simulink model "Model_turn"  (R2024a)
settings: Solver=VariableStepAuto  StartTime=0.0  StopTime=100  MaxStep=0.1  RelTol=1e-3
values from neighbouring files (symbols this model uses):
  c_SMA = 837.36    [params.m]
  Fmax_SMA = 10    [params.m]
  h_SMA = .3    (= 0.3)    [params.m]
  k_gn = m*g/0.01    (= 9810)    [contact3D_params.m]
  k_gt = m*g/0.1    (= 981)    [contact3D_params.m]
  m = 10    [contact3D_params.m]
  m_SMA = 0.0025    [params.m]
  max_SMA_Energy_J = 150    [params.m]
  mu_slide = 0.8    [contact3D_params.m]
  mu_stick = 0.9    [contact3D_params.m]
  n_segs = 10    [params.m]
  PWM_max = 0.35    [params.m]
  R_SMA = .08    (= 0.08)    [params.m]
  r_SMA2limb = 0.009    [params.m]
  swing_angle = swing_angles(i)    [params.m]
  T_amb = 23    [params.m]
  V_0 = 7    [params.m]
  v_gn_max = 0.03    [contact3D_params.m]
  v_gt_max = 0.03    [contact3D_params.m]
  vLimit = 0.01    [contact3D_params.m]
undefined symbols (not defined in the file or in its folder): Newton, Raphson, X, Y, Z
libraries: sm_lib x225, nesl_utility x185, simulink x24, simulink_extras x6
(part 15 of 16)

== system Model_turn/LIMB 1: Front LEFT/Limb 1/Right Ball Contact/3D Contact/Kinetic Friction Model ==
  note: Kinetic Friction Model
  note: Footpoint Determiner
  note: Sliding Limit Detector
  note: Normal Ground Friction
  note: Tangential Ground Friction
  vel [m/s m/s m/s] : Inport
  pos [m m m] : Inport  Port=2
  RefPt [m m m] : Inport  Port=3
  nVec [m m m] : Inport  Port=4
  Enable : EnablePort  StatesWhenEnabling=reset  ZeroCross=off
  Constant : Constant  Value=vLimit
  Constant1 : Constant  Value=[0 0 0 1]'
  Demux : Demux  Outputs=[3 1]
  FixPt Relational Operator : RelationalOperator  Operator=>  OutDataTypeStr=boolean  ZeroCross=off  InputSameDT=off
  Gain3 : Gain  Gain=k_gn
  Gain4 : Gain  Gain=1/v_gn_max
  Memory : Memory
  Mux1 : Mux  Inputs=2
  Mux2 : Mux  Inputs=2
  Negative : simulink/Logic and Bit Operations/Compare To Zero  relop=<  OutDataTypeStr=boolean
  Normal Axis Ground Force : Fcn  Expr="u(1)  *  (1-u(2)) * (u(2)<1)"
  Product : Product  RndMeth=Zero
  Product1 : Product  RndMeth=Zero
  Sum : Sum  Inputs=|+-
  Switch : Switch  Criteria=u2 > Threshold  Threshold=0.9*vLimit  SaturateOnIntegerOverflow=off  InputSameDT=off
      settings: AttributesFormatString=>%<Threshold>?
  Vector Norm : Subsystem
  d_n : DotProduct  OutDataTypeStr=Inherit: Inherit via internal rule
  qnVec : Sum  Inputs=-+
  reverse direction : Gain  Gain=-1
  sliding friction coefficient : Gain  Gain=mu_slide
  tVec : Product  Inputs=*/  RndMeth=Zero
  v_n : DotProduct  OutDataTypeStr=Inherit: Inherit via internal rule
  v_nVec : Product  RndMeth=Zero
  v_tVec : Sum  Inputs=-+|
  RefPtFP [m m m] : Outport  InitialOutput=[0 0 0]
      settings: AttributesFormatString=initial = '%<InitialOutput>'\nwhen disabled = '%<OutputWhenDisabled>'
  posFP [m m m] : Outport  Port=2  InitialOutput=[0 0 0]
      settings: AttributesFormatString=initial = '%<InitialOutput>'\nwhen disabled = '%<OutputWhenDisabled>'
  nVec FP [m m m] : Outport  Port=3  InitialOutput=0
      settings: AttributesFormatString=initial = '%<InitialOutput>'\nwhen disabled = '%<OutputWhenDisabled>'
  Stiction! : Outport  Port=4  OutputWhenDisabled=reset  InitialOutput=0
      settings: AttributesFormatString=initial = '%<InitialOutput>'\nwhen disabled = '%<OutputWhenDisabled>'
  F_t Slide [N N N] : Outport  Port=5  OutputWhenDisabled=reset  InitialOutput=[0 0 0]
      settings: AttributesFormatString=initial = '%<InitialOutput>'\nwhen disabled = '%<OutputWhenDisabled>'
  F_n Slide [N N N] : Outport  Port=6  OutputWhenDisabled=reset  InitialOutput=[0 0 0]
      settings: AttributesFormatString=initial = '%<InitialOutput>'\nwhen disabled = '%<OutputWhenDisabled>'
  wires:
  Normal Axis Ground Force/1 -> sliding friction coefficient/1, Product1/2
  Product/1 -> F_t Slide [N N N]/1
  FixPt Relational Operator/1 -> Stiction!/1
  Memory/1 -> FixPt Relational Operator/2
  Negative/1 -> FixPt Relational Operator/1, Memory/1
  Vector Norm/1(norm) -> Sum/1, Switch/2, Mux2/2
  Sum/1 -> Negative/1
  Constant/1 -> Sum/2
  Mux1/1 -> Normal Axis Ground Force/1
  Gain3/1 -> Mux1/1
  Gain4/1 -> Mux1/2
  nVec [m m m]/1 -> v_n/1, v_nVec/2, d_n/2, Product1/1, nVec FP [m m m]/1
  d_n/1 -> Gain3/1
  vel [m/s m/s m/s]/1 -> v_n/2, v_tVec/2
  v_n/1 -> Gain4/1, v_nVec/1
  v_nVec/1 -> v_tVec/1
  v_tVec/1 -> Vector Norm/1(vec), Mux2/1
  sliding friction coefficient/1 -> Product/1
  reverse direction/1 -> Product/2
  Product1/1 -> F_n Slide [N N N]/1
  tVec/1 -> reverse direction/1
  Constant1/1 -> Switch/3
  Mux2/1 -> Switch/1
  Switch/1 -> Demux/1
  Demux/2 -> tVec/2
  Demux/1 -> tVec/1
  pos [m m m]/1 -> posFP [m m m]/1, qnVec/1
  qnVec/1 -> d_n/1
  RefPt [m m m]/1 -> qnVec/2, RefPtFP [m m m]/1

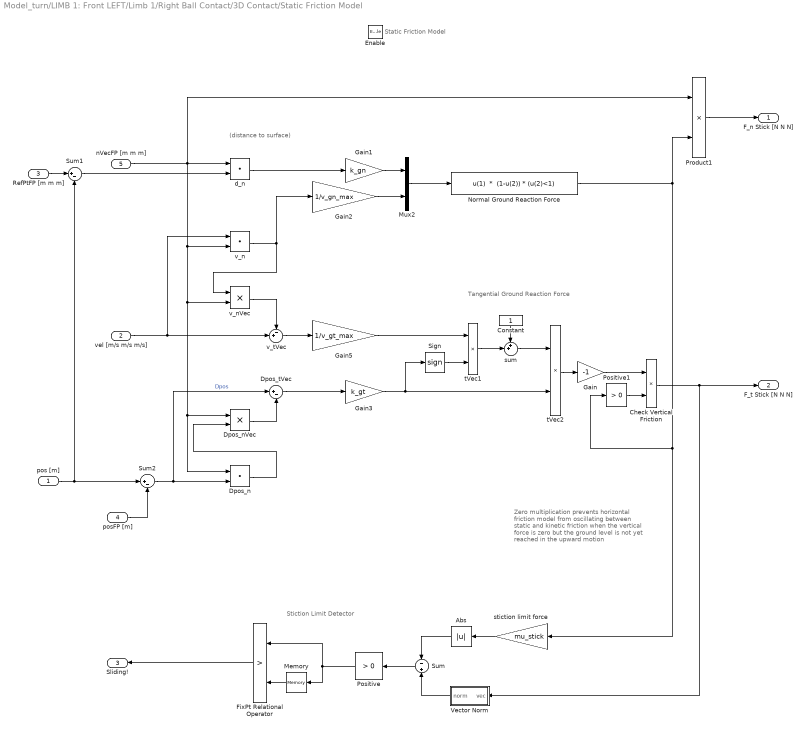
== system Model_turn/LIMB 1: Front LEFT/Limb 1/Right Ball Contact/3D Contact/Static Friction Model ==
  note: Stiction Limit Detector
  note: Static Friction Model
  note: Zero multiplication prevents
      | horizontal friction model from
      | oscillating between static and kinetic
      | friction when the vertical force is zero but
      | the ground level is not yet reached
      | in the upward motion
  note: (distance to
      | surface)
  note: Tangential Ground Reaction Force
  pos [m] : Inport
  vel [m/s m/s m/s] : Inport  Port=2
  RefPtFP [m m m] : Inport  Port=3
  posFP [m] : Inport  Port=4
  nVecFP [m m m] : Inport  Port=5
  Enable : EnablePort  StatesWhenEnabling=reset  ZeroCross=off
  Abs : Abs  SaturateOnIntegerOverflow=off
  Check Vertical Friction : Product  RndMeth=Zero
  Constant : Constant
  Dpos_n : DotProduct  OutDataTypeStr=Inherit: Inherit via internal rule
  Dpos_nVec : Product  RndMeth=Zero
  Dpos_tVec : Sum  Inputs=|+-
  FixPt Relational Operator : RelationalOperator  Operator=>  OutDataTypeStr=boolean  ZeroCross=off  InputSameDT=off
  Gain : Gain  Gain=-1
  Gain1 : Gain  Gain=k_gn
  Gain2 : Gain  Gain=1/v_gn_max
  Gain3 : Gain  Gain=k_gt
  Gain5 : Gain  Gain=1/v_gt_max
  Memory : Memory
  Mux2 : Mux  Inputs=2
  Normal Ground Reaction Force : Fcn  Expr="u(1)  *  (1-u(2)) * (u(2)<1)"
  Positive : simulink/Logic and Bit Operations/Compare To Zero  relop=>  OutDataTypeStr=boolean
  Positive1 : simulink/Logic and Bit Operations/Compare To Zero  relop=>  OutDataTypeStr=boolean
  Product1 : Product  RndMeth=Zero
  Sign : Signum  ZeroCross=off
  Sum : Sum  Inputs=-+
  Sum1 : Sum  Inputs=|+-
  Sum2 : Sum  Inputs=|+-
  Vector Norm : Subsystem
  d_n : DotProduct  OutDataTypeStr=Inherit: Inherit via internal rule
  stiction limit force : Gain  Gain=mu_stick
  sum : Sum  Inputs=++|
  tVec1 : Product  Inputs=**  RndMeth=Zero
  tVec2 : Product  Inputs=**  RndMeth=Zero
  v_n : DotProduct  OutDataTypeStr=Inherit: Inherit via internal rule
  v_nVec : Product  RndMeth=Zero
  v_tVec : Sum  Inputs=-+|
  F_n Stick [N N N] : Outport  OutputWhenDisabled=reset  InitialOutput=[0 0 0]
      settings: AttributesFormatString=initial = '%<InitialOutput>'\nwhen disabled = '%<OutputWhenDisabled>'
  F_t Stick [N N N] : Outport  Port=2  OutputWhenDisabled=reset  InitialOutput=[0 0 0]
      settings: AttributesFormatString=when disabled: %<OutputWhenDisabled>\ninitial: %<InitialOutput>
  Sliding! : Outport  Port=3  OutputWhenDisabled=reset  InitialOutput=0
      settings: AttributesFormatString=when disabled: %<OutputWhenDisabled>\ninitial: %<InitialOutput>
  wires:
  Sum/1 -> Positive/1
  Memory/1 -> FixPt Relational Operator/2
  Positive/1 -> FixPt Relational Operator/1, Memory/1
  FixPt Relational Operator/1 -> Sliding!/1
  Abs/1 -> Sum/1
  stiction limit force/1 -> Abs/1
  Positive1/1 -> Check Vertical Friction/2
  Check Vertical Friction/1 -> Vector Norm/1(vec), F_t Stick [N N N]/1
  Normal Ground Reaction Force/1 -> Product1/2, stiction limit force/1, Positive1/1
  Mux2/1 -> Normal Ground Reaction Force/1
  Gain1/1 -> Mux2/1
  Gain2/1 -> Mux2/2
  nVecFP [m m m]/1 -> d_n/1, v_n/2, Dpos_n/1, Dpos_nVec/1, v_nVec/2, Product1/1
  d_n/1 -> Gain1/1
  vel [m/s m/s m/s]/1 -> v_tVec/2, v_n/1
  v_n/1 -> v_nVec/1, Gain2/1
  v_nVec/1 -> v_tVec/1
  v_tVec/1 -> Gain5/1
  Product1/1 -> F_n Stick [N N N]/1
  pos [m]/1 -> Sum2/1, Sum1/2
  posFP [m]/1 -> Sum2/2
  Sum2/1 -> Dpos_n/2, Dpos_tVec/1  "Dpos"
  Dpos_n/1 -> Dpos_nVec/2
  Dpos_nVec/1 -> Dpos_tVec/2
  Dpos_tVec/1 -> Gain3/1
  Gain3/1 -> Sign/1, tVec2/2
  Sign/1 -> tVec1/2
  tVec1/1 -> sum/2
  Constant/1 -> sum/1
  sum/1 -> tVec2/1
  tVec2/1 -> Gain/1
  Gain/1 -> Check Vertical Friction/1
  Vector Norm/1(norm) -> Sum/2
  RefPtFP [m m m]/1 -> Sum1/1
  Sum1/1 -> d_n/2
  Gain5/1 -> tVec1/1

== system Model_turn/LIMB 1: Front RIGHT/Limb 1/Right Ball Contact/3D Contact/Friction Switch ==
  note: Static/Kinetic Friction Switch
  Slide! : Inport
  Stick! : Inport  Port=2
  Memory : Memory
  S-R Flip-Flop : simulink_extras/Flip Flops/S-R Flip-Flop  initial_condition=0
  Terminator : Terminator
  Stiction : Outport
  wires:
  S-R Flip-Flop/1 -> Memory/1
  S-R Flip-Flop/2 -> Terminator/1
  Stick!/1 -> S-R Flip-Flop/1
  Slide!/1 -> S-R Flip-Flop/2
  Memory/1 -> Stiction/1

== system Model_turn/LIMB 1: Front RIGHT/Limb 1/Right Ball Contact/3D Contact/Kinetic Friction Model ==
  note: Kinetic Friction Model
  note: Footpoint Determiner
  note: Sliding Limit Detector
  note: Normal Ground Friction
  note: Tangential Ground Friction
  vel [m/s m/s m/s] : Inport
  pos [m m m] : Inport  Port=2
  RefPt [m m m] : Inport  Port=3
  nVec [m m m] : Inport  Port=4
  Enable : EnablePort  StatesWhenEnabling=reset  ZeroCross=off
  Constant : Constant  Value=vLimit
  Constant1 : Constant  Value=[0 0 0 1]'
  Demux : Demux  Outputs=[3 1]
  FixPt Relational Operator : RelationalOperator  Operator=>  OutDataTypeStr=boolean  ZeroCross=off  InputSameDT=off
  Gain3 : Gain  Gain=k_gn
  Gain4 : Gain  Gain=1/v_gn_max
  Memory : Memory
  Mux1 : Mux  Inputs=2
  Mux2 : Mux  Inputs=2
  Negative : simulink/Logic and Bit Operations/Compare To Zero  relop=<  OutDataTypeStr=boolean
  Normal Axis Ground Force : Fcn  Expr="u(1)  *  (1-u(2)) * (u(2)<1)"
  Product : Product  RndMeth=Zero
  Product1 : Product  RndMeth=Zero
  Sum : Sum  Inputs=|+-
  Switch : Switch  Criteria=u2 > Threshold  Threshold=0.9*vLimit  SaturateOnIntegerOverflow=off  InputSameDT=off
      settings: AttributesFormatString=>%<Threshold>?
  Vector Norm : Subsystem
  d_n : DotProduct  OutDataTypeStr=Inherit: Inherit via internal rule
  qnVec : Sum  Inputs=-+
  reverse direction : Gain  Gain=-1
  sliding friction coefficient : Gain  Gain=mu_slide
  tVec : Product  Inputs=*/  RndMeth=Zero
  v_n : DotProduct  OutDataTypeStr=Inherit: Inherit via internal rule
  v_nVec : Product  RndMeth=Zero
  v_tVec : Sum  Inputs=-+|
  RefPtFP [m m m] : Outport  InitialOutput=[0 0 0]
      settings: AttributesFormatString=initial = '%<InitialOutput>'\nwhen disabled = '%<OutputWhenDisabled>'
  posFP [m m m] : Outport  Port=2  InitialOutput=[0 0 0]
      settings: AttributesFormatString=initial = '%<InitialOutput>'\nwhen disabled = '%<OutputWhenDisabled>'
  nVec FP [m m m] : Outport  Port=3  InitialOutput=0
      settings: AttributesFormatString=initial = '%<InitialOutput>'\nwhen disabled = '%<OutputWhenDisabled>'
  Stiction! : Outport  Port=4  OutputWhenDisabled=reset  InitialOutput=0
      settings: AttributesFormatString=initial = '%<InitialOutput>'\nwhen disabled = '%<OutputWhenDisabled>'
  F_t Slide [N N N] : Outport  Port=5  OutputWhenDisabled=reset  InitialOutput=[0 0 0]
      settings: AttributesFormatString=initial = '%<InitialOutput>'\nwhen disabled = '%<OutputWhenDisabled>'
  F_n Slide [N N N] : Outport  Port=6  OutputWhenDisabled=reset  InitialOutput=[0 0 0]
      settings: AttributesFormatString=initial = '%<InitialOutput>'\nwhen disabled = '%<OutputWhenDisabled>'
  wires:
  Normal Axis Ground Force/1 -> sliding friction coefficient/1, Product1/2
  Product/1 -> F_t Slide [N N N]/1
  FixPt Relational Operator/1 -> Stiction!/1
  Memory/1 -> FixPt Relational Operator/2
  Negative/1 -> FixPt Relational Operator/1, Memory/1
  Vector Norm/1(norm) -> Sum/1, Switch/2, Mux2/2
  Sum/1 -> Negative/1
  Constant/1 -> Sum/2
  Mux1/1 -> Normal Axis Ground Force/1
  Gain3/1 -> Mux1/1
  Gain4/1 -> Mux1/2
  nVec [m m m]/1 -> v_n/1, v_nVec/2, d_n/2, Product1/1, nVec FP [m m m]/1
  d_n/1 -> Gain3/1
  vel [m/s m/s m/s]/1 -> v_n/2, v_tVec/2
  v_n/1 -> Gain4/1, v_nVec/1
  v_nVec/1 -> v_tVec/1
  v_tVec/1 -> Vector Norm/1(vec), Mux2/1
  sliding friction coefficient/1 -> Product/1
  reverse direction/1 -> Product/2
  Product1/1 -> F_n Slide [N N N]/1
  tVec/1 -> reverse direction/1
  Constant1/1 -> Switch/3
  Mux2/1 -> Switch/1
  Switch/1 -> Demux/1
  Demux/2 -> tVec/2
  Demux/1 -> tVec/1
  pos [m m m]/1 -> posFP [m m m]/1, qnVec/1
  qnVec/1 -> d_n/1
  RefPt [m m m]/1 -> qnVec/2, RefPtFP [m m m]/1

== system Model_turn/LIMB 1: Front RIGHT/Limb 1/Right Ball Contact/3D Contact/Static Friction Model ==
  note: Stiction Limit Detector
  note: Static Friction Model
  note: Zero multiplication prevents
      | horizontal friction model from
      | oscillating between static and kinetic
      | friction when the vertical force is zero but
      | the ground level is not yet reached
      | in the upward motion
  note: (distance to
      | surface)
  note: Tangential Ground Reaction Force
  pos [m] : Inport
  vel [m/s m/s m/s] : Inport  Port=2
  RefPtFP [m m m] : Inport  Port=3
  posFP [m] : Inport  Port=4
  nVecFP [m m m] : Inport  Port=5
  Enable : EnablePort  StatesWhenEnabling=reset  ZeroCross=off
  Abs : Abs  SaturateOnIntegerOverflow=off
  Check Vertical Friction : Product  RndMeth=Zero
  Constant : Constant
  Dpos_n : DotProduct  OutDataTypeStr=Inherit: Inherit via internal rule
  Dpos_nVec : Product  RndMeth=Zero
  Dpos_tVec : Sum  Inputs=|+-
  FixPt Relational Operator : RelationalOperator  Operator=>  OutDataTypeStr=boolean  ZeroCross=off  InputSameDT=off
  Gain : Gain  Gain=-1
  Gain1 : Gain  Gain=k_gn
  Gain2 : Gain  Gain=1/v_gn_max
  Gain3 : Gain  Gain=k_gt
  Gain5 : Gain  Gain=1/v_gt_max
  Memory : Memory
  Mux2 : Mux  Inputs=2
  Normal Ground Reaction Force : Fcn  Expr="u(1)  *  (1-u(2)) * (u(2)<1)"
  Positive : simulink/Logic and Bit Operations/Compare To Zero  relop=>  OutDataTypeStr=boolean
  Positive1 : simulink/Logic and Bit Operations/Compare To Zero  relop=>  OutDataTypeStr=boolean
  Product1 : Product  RndMeth=Zero
  Sign : Signum  ZeroCross=off
  Sum : Sum  Inputs=-+
  Sum1 : Sum  Inputs=|+-
  Sum2 : Sum  Inputs=|+-
  Vector Norm : Subsystem
  d_n : DotProduct  OutDataTypeStr=Inherit: Inherit via internal rule
  stiction limit force : Gain  Gain=mu_stick
  sum : Sum  Inputs=++|
  tVec1 : Product  Inputs=**  RndMeth=Zero
  tVec2 : Product  Inputs=**  RndMeth=Zero
  v_n : DotProduct  OutDataTypeStr=Inherit: Inherit via internal rule
  v_nVec : Product  RndMeth=Zero
  v_tVec : Sum  Inputs=-+|
  F_n Stick [N N N] : Outport  OutputWhenDisabled=reset  InitialOutput=[0 0 0]
      settings: AttributesFormatString=initial = '%<InitialOutput>'\nwhen disabled = '%<OutputWhenDisabled>'
  F_t Stick [N N N] : Outport  Port=2  OutputWhenDisabled=reset  InitialOutput=[0 0 0]
      settings: AttributesFormatString=when disabled: %<OutputWhenDisabled>\ninitial: %<InitialOutput>
  Sliding! : Outport  Port=3  OutputWhenDisabled=reset  InitialOutput=0
      settings: AttributesFormatString=when disabled: %<OutputWhenDisabled>\ninitial: %<InitialOutput>
  wires:
  Sum/1 -> Positive/1
  Memory/1 -> FixPt Relational Operator/2
  Positive/1 -> FixPt Relational Operator/1, Memory/1
  FixPt Relational Operator/1 -> Sliding!/1
  Abs/1 -> Sum/1
  stiction limit force/1 -> Abs/1
  Positive1/1 -> Check Vertical Friction/2
  Check Vertical Friction/1 -> Vector Norm/1(vec), F_t Stick [N N N]/1
  Normal Ground Reaction Force/1 -> Product1/2, stiction limit force/1, Positive1/1
  Mux2/1 -> Normal Ground Reaction Force/1
  Gain1/1 -> Mux2/1
  Gain2/1 -> Mux2/2
  nVecFP [m m m]/1 -> d_n/1, v_n/2, Dpos_n/1, Dpos_nVec/1, v_nVec/2, Product1/1
  d_n/1 -> Gain1/1
  vel [m/s m/s m/s]/1 -> v_tVec/2, v_n/1
  v_n/1 -> v_nVec/1, Gain2/1
  v_nVec/1 -> v_tVec/1
  v_tVec/1 -> Gain5/1
  Product1/1 -> F_n Stick [N N N]/1
  pos [m]/1 -> Sum2/1, Sum1/2
  posFP [m]/1 -> Sum2/2
  Sum2/1 -> Dpos_n/2, Dpos_tVec/1  "Dpos"
  Dpos_n/1 -> Dpos_nVec/2
  Dpos_nVec/1 -> Dpos_tVec/2
  Dpos_tVec/1 -> Gain3/1
  Gain3/1 -> Sign/1, tVec2/2
  Sign/1 -> tVec1/2
  tVec1/1 -> sum/2
  Constant/1 -> sum/1
  sum/1 -> tVec2/1
  tVec2/1 -> Gain/1
  Gain/1 -> Check Vertical Friction/1
  Vector Norm/1(norm) -> Sum/2
  RefPtFP [m m m]/1 -> Sum1/1
  Sum1/1 -> d_n/2
  Gain5/1 -> tVec1/1

== system Model_turn/LIMB 1: Back LEFT/Limb 1/Right Ball Contact/3D Contact/Kinetic Friction Model/Vector Norm ==
  vec : Inport
  Sqrt : Sqrt  OutputSignalType=real  AlgorithmType=Newton-Raphson
  Squares : Math  Operator=square  SignedPower=on  OutputSignalType=real
  Sum of Elements : Sum  Inputs=+
  norm : Outport
  wires:
  vec/1 -> Squares/1
  Sqrt/1 -> norm/1
  Sum of Elements/1 -> Sqrt/1
  Squares/1 -> Sum of Elements/1

== system Model_turn/LIMB 1: Back LEFT/Limb 1/Right Ball Contact/3D Contact/Static Friction Model/Vector Norm ==
  vec : Inport
  Sqrt : Sqrt  OutputSignalType=real  AlgorithmType=Newton-Raphson
  Squares : Math  Operator=square  SignedPower=on  OutputSignalType=real
  Sum of Elements : Sum  Inputs=+
  norm : Outport
  wires:
  vec/1 -> Squares/1
  Sqrt/1 -> norm/1
  Sum of Elements/1 -> Sqrt/1
  Squares/1 -> Sum of Elements/1

== system Model_turn/LIMB 1: Back RIGHT/Limb 1/Right Ball Contact/3D Contact/Kinetic Friction Model/Vector Norm ==
  vec : Inport
  Sqrt : Sqrt  OutputSignalType=real  AlgorithmType=Newton-Raphson
  Squares : Math  Operator=square  SignedPower=on  OutputSignalType=real
  Sum of Elements : Sum  Inputs=+
  norm : Outport
  wires:
  vec/1 -> Squares/1
  Sqrt/1 -> norm/1
  Sum of Elements/1 -> Sqrt/1
  Squares/1 -> Sum of Elements/1

== system Model_turn/LIMB 1: Back RIGHT/Limb 1/Right Ball Contact/3D Contact/Static Friction Model/Vector Norm ==
  vec : Inport
  Sqrt : Sqrt  OutputSignalType=real  AlgorithmType=Newton-Raphson
  Squares : Math  Operator=square  SignedPower=on  OutputSignalType=real
  Sum of Elements : Sum  Inputs=+
  norm : Outport
  wires:
  vec/1 -> Squares/1
  Sqrt/1 -> norm/1
  Sum of Elements/1 -> Sqrt/1
  Squares/1 -> Sum of Elements/1

== system Model_turn/LIMB 1: Center LEFT/Limb 1/Right Ball Contact/3D Contact/Kinetic Friction Model/Vector Norm ==
  vec : Inport
  Sqrt : Sqrt  OutputSignalType=real  AlgorithmType=Newton-Raphson
  Squares : Math  Operator=square  SignedPower=on  OutputSignalType=real
  Sum of Elements : Sum  Inputs=+
  norm : Outport
  wires:
  vec/1 -> Squares/1
  Sqrt/1 -> norm/1
  Sum of Elements/1 -> Sqrt/1
  Squares/1 -> Sum of Elements/1

== system Model_turn/LIMB 1: Center LEFT/Limb 1/Right Ball Contact/3D Contact/Static Friction Model/Vector Norm ==
  vec : Inport
  Sqrt : Sqrt  OutputSignalType=real  AlgorithmType=Newton-Raphson
  Squares : Math  Operator=square  SignedPower=on  OutputSignalType=real
  Sum of Elements : Sum  Inputs=+
  norm : Outport
  wires:
  vec/1 -> Squares/1
  Sqrt/1 -> norm/1
  Sum of Elements/1 -> Sqrt/1
  Squares/1 -> Sum of Elements/1

== system Model_turn/LIMB 1: Center RIGHT/Limb 1/Right Ball Contact/3D Contact/Kinetic Friction Model/Vector Norm ==
  vec : Inport
  Sqrt : Sqrt  OutputSignalType=real  AlgorithmType=Newton-Raphson
  Squares : Math  Operator=square  SignedPower=on  OutputSignalType=real
  Sum of Elements : Sum  Inputs=+
  norm : Outport
  wires:
  vec/1 -> Squares/1
  Sqrt/1 -> norm/1
  Sum of Elements/1 -> Sqrt/1
  Squares/1 -> Sum of Elements/1

== system Model_turn/LIMB 1: Center RIGHT/Limb 1/Right Ball Contact/3D Contact/Static Friction Model/Vector Norm ==
  vec : Inport
  Sqrt : Sqrt  OutputSignalType=real  AlgorithmType=Newton-Raphson
  Squares : Math  Operator=square  SignedPower=on  OutputSignalType=real
  Sum of Elements : Sum  Inputs=+
  norm : Outport
  wires:
  vec/1 -> Squares/1
  Sqrt/1 -> norm/1
  Sum of Elements/1 -> Sqrt/1
  Squares/1 -> Sum of Elements/1

== system Model_turn/LIMB 1: Front LEFT/Limb 1/Right Ball Contact/3D Contact/Kinetic Friction Model/Vector Norm ==
  vec : Inport
  Sqrt : Sqrt  OutputSignalType=real  AlgorithmType=Newton-Raphson
  Squares : Math  Operator=square  SignedPower=on  OutputSignalType=real
  Sum of Elements : Sum  Inputs=+
  norm : Outport
  wires:
  vec/1 -> Squares/1
  Sqrt/1 -> norm/1
  Sum of Elements/1 -> Sqrt/1
  Squares/1 -> Sum of Elements/1

== system Model_turn/LIMB 1: Front LEFT/Limb 1/Right Ball Contact/3D Contact/Static Friction Model/Vector Norm ==
  vec : Inport
  Sqrt : Sqrt  OutputSignalType=real  AlgorithmType=Newton-Raphson
  Squares : Math  Operator=square  SignedPower=on  OutputSignalType=real
  Sum of Elements : Sum  Inputs=+
  norm : Outport
  wires:
  vec/1 -> Squares/1
  Sqrt/1 -> norm/1
  Sum of Elements/1 -> Sqrt/1
  Squares/1 -> Sum of Elements/1

== system Model_turn/LIMB 1: Front RIGHT/Limb 1/Right Ball Contact/3D Contact/Kinetic Friction Model/Vector Norm ==
  vec : Inport
  Sqrt : Sqrt  OutputSignalType=real  AlgorithmType=Newton-Raphson
  Squares : Math  Operator=square  SignedPower=on  OutputSignalType=real
  Sum of Elements : Sum  Inputs=+
  norm : Outport
  wires:
  vec/1 -> Squares/1
  Sqrt/1 -> norm/1
  Sum of Elements/1 -> Sqrt/1
  Squares/1 -> Sum of Elements/1

== system Model_turn/LIMB 1: Front RIGHT/Limb 1/Right Ball Contact/3D Contact/Static Friction Model/Vector Norm ==
  vec : Inport
  Sqrt : Sqrt  OutputSignalType=real  AlgorithmType=Newton-Raphson
  Squares : Math  Operator=square  SignedPower=on  OutputSignalType=real
  Sum of Elements : Sum  Inputs=+
  norm : Outport
  wires:
  vec/1 -> Squares/1
  Sqrt/1 -> norm/1
  Sum of Elements/1 -> Sqrt/1
  Squares/1 -> Sum of Elements/1

== matlab function Model_turn/LIMB 1: Back RIGHT/Limb 1/MATLAB Function2 ==
  data: R input; roll_deg output; pitch_deg output; yaw_deg output
function [roll_deg, pitch_deg, yaw_deg] = orientation_to_plane_angles(R)
    roll = atan2(R(3,2), R(3,3));
    pitch = asin(-R(3,1));
    yaw = atan2(R(2,1), R(1,1));
    % Convert angles from radians to degrees
    roll_deg = rad2deg(roll);
    pitch_deg = rad2deg(pitch);
    yaw_deg = rad2deg(yaw);

end

== matlab function Model_turn/LIMB 1: Back RIGHT/Limb 1/SMA1 F(V)/F(T) ==
  data: T input; F output; Fmax_SMA input
function F = fcn(T, Fmax_SMA)

% INPUT: Temperature (C), max SMA force
% OUTPUT: Force [N]

% Based around T_transition = 90C

% THOS WHOLE RELATIONSHIP NEEDS IMPROVEMENT, LOOSELY BASED ON fig 6b from:
% https://link.springer.com/article/10.1007/s11340-024-01059-9 and 
% https://www.dynalloy.com/pdfs/TCF1140_2.pdf
if T>110
    F = Fmax_SMA;
elseif T>95
    F = Fmax_SMA - 0.2*Fmax_SMA * ((110-T)/15);
elseif T>85
    F = 0.8*Fmax_SMA - 0.55*Fmax_SMA * ((95-T)/10);
else
    F = 0.25*Fmax_SMA - 0.25*Fmax_SMA * ((85-T)/50);
end

== matlab function Model_turn/LIMB 1: Back RIGHT/Limb 1/SMA2 F(V)/F(T) ==
  data: T input; F output; Fmax_SMA input
function F = fcn(T, Fmax_SMA)

% INPUT: Temperature (C), max SMA force
% OUTPUT: Force [N]

% Based around T_transition = 90C

% THOS WHOLE RELATIONSHIP NEEDS IMPROVEMENT, LOOSELY BASED ON fig 6b from:
% https://link.springer.com/article/10.1007/s11340-024-01059-9 and 
% https://www.dynalloy.com/pdfs/TCF1140_2.pdf
if T>110
    F = Fmax_SMA;
elseif T>95
    F = Fmax_SMA - 0.2*Fmax_SMA * ((110-T)/15);
elseif T>85
    F = 0.8*Fmax_SMA - 0.55*Fmax_SMA * ((95-T)/10);
else
    F = 0.25*Fmax_SMA - 0.25*Fmax_SMA * ((85-T)/50);
end

== matlab function Model_turn/LIMB 1: Back RIGHT/Limb 1/SMA3 F(V)/F(T) ==
  data: T input; F output; Fmax_SMA input
function F = fcn(T, Fmax_SMA)

% INPUT: Temperature (C), max SMA force
% OUTPUT: Force [N]

% Based around T_transition = 90C

% THOS WHOLE RELATIONSHIP NEEDS IMPROVEMENT, LOOSELY BASED ON fig 6b from:
% https://link.springer.com/article/10.1007/s11340-024-01059-9 and 
% https://www.dynalloy.com/pdfs/TCF1140_2.pdf
if T>110
    F = Fmax_SMA;
elseif T>95
    F = Fmax_SMA - 0.2*Fmax_SMA * ((110-T)/15);
elseif T>85
    F = 0.8*Fmax_SMA - 0.55*Fmax_SMA * ((95-T)/10);
else
    F = 0.25*Fmax_SMA - 0.25*Fmax_SMA * ((85-T)/50);
end

== matlab function Model_turn/LIMB 1: Back RIGHT/Limb 1/SMA4 F(V)/F(T) ==
  data: T input; F output; Fmax_SMA input
function F = fcn(T, Fmax_SMA)

% INPUT: Temperature (C), max SMA force
% OUTPUT: Force [N]

% Based around T_transition = 90C

% THOS WHOLE RELATIONSHIP NEEDS IMPROVEMENT, LOOSELY BASED ON fig 6b from:
% https://link.springer.com/article/10.1007/s11340-024-01059-9 and 
% https://www.dynalloy.com/pdfs/TCF1140_2.pdf
if T>110
    F = Fmax_SMA;
elseif T>95
    F = Fmax_SMA - 0.2*Fmax_SMA * ((110-T)/15);
elseif T>85
    F = 0.8*Fmax_SMA - 0.55*Fmax_SMA * ((95-T)/10);
else
    F = 0.25*Fmax_SMA - 0.25*Fmax_SMA * ((85-T)/50);
end

== matlab function Model_turn/LIMB 1: Back RIGHT/PID CONTROLLER ==
  data: eX input; deX input; seX input; D1 output; eY input; D2 output; D3 output; D4 output; deY input; seY input; PWM_max input
function [D1, D2, D3, D4] = fcn(eX, deX, seX, eY, deY, seY, PWM_max)

    % INPUT: errors and derivatives about -x and -y axes, max PWM
    % OUTPUT: Duty Cycles:

    kp = 0.5;
    kd = 0;
    ki = 0.05;

    D1 = 0; D2 = 0; D3 = 0; D4 = 0;

    if eX > 0.5
        D1 = min((kp*eX + kd*deX + ki*seX), PWM_max);
    elseif eX < -0.5
        D2 = min((kp*-eX + kd*-deX + ki*-seX), PWM_max);
    end

    if eY > 0.5
        D3 = min((kp*eY + kd*deY + ki*seY), PWM_max);
    elseif eY < -0.5
        D4 = min((kp*-eY + kd*-deY + ki*-seY), PWM_max);
    end

== matlab function Model_turn/LIMB 1: Front LEFT/BANG-BANG CONTROLLER ==
  data: theta_X input; D1 output; theta_Y input; D2 output; D3 output; D4 output; Target_X input; Target_Y input; PWM_max input
function [D1, D2, D3, D4] = fcn(theta_X, theta_Y, Target_X, Target_Y, PWM_max)

    % INPUT: Rotations about -X and -Y axes, Target angles, max PWM
    % OUTPUT: Duty Cycles:
    %   D1: +X rotation
    %   D2: -X rotation
    %   D3: +Y rotation
    %   D4: -Y rotation

    X_err = Target_X - theta_X;
    Y_err = Target_Y - theta_Y;

    D1 = 0; D2 = 0; D3 = 0; D4 = 0;

    if X_err > 5
        D1 = PWM_max;
    elseif X_err > 1
        D1 = PWM_max / 1.5;
    elseif X_err < -5
        D2 = PWM_max;
    elseif X_err < -1
        D2 = PWM_max / 1.5;
    end

    if Y_err > 5
        D3 = PWM_max;
    elseif Y_err > 1
        D3 = PWM_max / 1.5;
    elseif Y_err < -5
        D4 = PWM_max;
    elseif Y_err < -1
        D4 = PWM_max / 1.5;
    end

== matlab function Model_turn/LIMB 1: Front LEFT/Limb 1/MATLAB Function1 ==
  data: R input; alpha_xz output; alpha_yz output; alpha_xy output
function [alpha_xz, alpha_yz, alpha_xy] = orientation_to_plane_angles(R)
% ORIENTATION_TO_PLANE_ANGLES Convert orientation to angle projections on XZ, YZ, XY planes
%   Inputs:
%       R - Rotation Matrix
%   Outputs:
%       alpha_xz - Angle in radians on the XZ-plane
%       alpha_yz - Angle in radians on the YZ-plane
%       alpha_xy - Angle in radians on the XY-plane
    
    % Define the local forward vector (local Z-axis)
    v_local = [0; 0; 1];
    
    % Transform to global coordinates
    v_global = R * v_local;
    
    % Projection onto XZ-plane
    v_xz = [v_global(1); 0; v_global(3)];
    alpha_xz = rad2deg(-(atan2(v_xz(3), v_xz(1)) - pi/2));
    
    % Projection onto YZ-plane
    v_yz = [0; v_global(2); v_global(3)];
    alpha_yz = rad2deg(atan2(v_yz(3), v_yz(2)) - pi/2);
    
    % Projection onto XY-plane
    v_xy = [v_global(1); v_global(2); 0];
    alpha_xy = rad2deg(atan2(v_xy(2), v_xy(1)) + pi/4);
end

== matlab function Model_turn/LIMB 1: Front LEFT/Limb 1/SMA1 F(V)/F(T) ==
  data: T input; F output; Fmax_SMA input
function F = fcn(T, Fmax_SMA)

% INPUT: Temperature (C), max SMA force
% OUTPUT: Force [N]

% Based around T_transition = 90C

% THOS WHOLE RELATIONSHIP NEEDS IMPROVEMENT, LOOSELY BASED ON fig 6b from:
% https://link.springer.com/article/10.1007/s11340-024-01059-9 and 
% https://www.dynalloy.com/pdfs/TCF1140_2.pdf
if T>110
    F = Fmax_SMA;
elseif T>95
    F = Fmax_SMA - 0.2*Fmax_SMA * ((110-T)/15);
elseif T>85
    F = 0.8*Fmax_SMA - 0.55*Fmax_SMA * ((95-T)/10);
else
    F = 0.25*Fmax_SMA - 0.25*Fmax_SMA * ((85-T)/50);
end

== matlab function Model_turn/LIMB 1: Front LEFT/Limb 1/SMA2 F(V)/F(T) ==
  data: T input; F output; Fmax_SMA input
function F = fcn(T, Fmax_SMA)

% INPUT: Temperature (C), max SMA force
% OUTPUT: Force [N]

% Based around T_transition = 90C

% THOS WHOLE RELATIONSHIP NEEDS IMPROVEMENT, LOOSELY BASED ON fig 6b from:
% https://link.springer.com/article/10.1007/s11340-024-01059-9 and 
% https://www.dynalloy.com/pdfs/TCF1140_2.pdf
if T>110
    F = Fmax_SMA;
elseif T>95
    F = Fmax_SMA - 0.2*Fmax_SMA * ((110-T)/15);
elseif T>85
    F = 0.8*Fmax_SMA - 0.55*Fmax_SMA * ((95-T)/10);
else
    F = 0.25*Fmax_SMA - 0.25*Fmax_SMA * ((85-T)/50);
end

== matlab function Model_turn/LIMB 1: Front LEFT/Limb 1/SMA3 F(V)/F(T) ==
  data: T input; F output; Fmax_SMA input
function F = fcn(T, Fmax_SMA)

% INPUT: Temperature (C), max SMA force
% OUTPUT: Force [N]

% Based around T_transition = 90C

% THOS WHOLE RELATIONSHIP NEEDS IMPROVEMENT, LOOSELY BASED ON fig 6b from:
% https://link.springer.com/article/10.1007/s11340-024-01059-9 and 
% https://www.dynalloy.com/pdfs/TCF1140_2.pdf
if T>110
    F = Fmax_SMA;
elseif T>95
    F = Fmax_SMA - 0.2*Fmax_SMA * ((110-T)/15);
elseif T>85
    F = 0.8*Fmax_SMA - 0.55*Fmax_SMA * ((95-T)/10);
else
    F = 0.25*Fmax_SMA - 0.25*Fmax_SMA * ((85-T)/50);
end

== matlab function Model_turn/LIMB 1: Front LEFT/Limb 1/SMA4 F(V)/F(T) ==
  data: T input; F output; Fmax_SMA input
function F = fcn(T, Fmax_SMA)

% INPUT: Temperature (C), max SMA force
% OUTPUT: Force [N]

% Based around T_transition = 90C

% THOS WHOLE RELATIONSHIP NEEDS IMPROVEMENT, LOOSELY BASED ON fig 6b from:
% https://link.springer.com/article/10.1007/s11340-024-01059-9 and 
% https://www.dynalloy.com/pdfs/TCF1140_2.pdf
if T>110
    F = Fmax_SMA;
elseif T>95
    F = Fmax_SMA - 0.2*Fmax_SMA * ((110-T)/15);
elseif T>85
    F = 0.8*Fmax_SMA - 0.55*Fmax_SMA * ((95-T)/10);
else
    F = 0.25*Fmax_SMA - 0.25*Fmax_SMA * ((85-T)/50);
end

== matlab function Model_turn/LIMB 1: Front LEFT/PID CONTROLLER ==
  data: eX input; deX input; seX input; D1 output; eY input; D2 output; D3 output; D4 output; deY input; seY input; PWM_max input
function [D1, D2, D3, D4] = fcn(eX, deX, seX, eY, deY, seY, PWM_max)

    % INPUT: errors and derivatives about -x and -y axes, max PWM
    % OUTPUT: Duty Cycles:

    kp = 0.5;
    kd = 0;
    ki = 0.05;

    D1 = 0; D2 = 0; D3 = 0; D4 = 0;

    if eX > 0.5
        D1 = min((kp*eX + kd*deX + ki*seX), PWM_max);
    elseif eX < -0.5
        D2 = min((kp*-eX + kd*-deX + ki*-seX), PWM_max);
    end

    if eY > 0.5
        D3 = min((kp*eY + kd*deY + ki*seY), PWM_max);
    elseif eY < -0.5
        D4 = min((kp*-eY + kd*-deY + ki*-seY), PWM_max);
    end

== matlab function Model_turn/LIMB 1: Back LEFT/BANG-BANG CONTROLLER ==
  data: theta_X input; D1 output; theta_Y input; D2 output; D3 output; D4 output; Target_X input; Target_Y input; PWM_max input
function [D1, D2, D3, D4] = fcn(theta_X, theta_Y, Target_X, Target_Y, PWM_max)

    % INPUT: Rotations about -X and -Y axes, Target angles, max PWM
    % OUTPUT: Duty Cycles:
    %   D1: +X rotation
    %   D2: -X rotation
    %   D3: +Y rotation
    %   D4: -Y rotation

    X_err = Target_X - theta_X;
    Y_err = Target_Y - theta_Y;

    D1 = 0; D2 = 0; D3 = 0; D4 = 0;

    if X_err > 5
        D1 = PWM_max;
    elseif X_err > 1
        D1 = PWM_max / 1.5;
    elseif X_err < -5
        D2 = PWM_max;
    elseif X_err < -1
        D2 = PWM_max / 1.5;
    end

    if Y_err > 5
        D3 = PWM_max;
    elseif Y_err > 1
        D3 = PWM_max / 1.5;
    elseif Y_err < -5
        D4 = PWM_max;
    elseif Y_err < -1
        D4 = PWM_max / 1.5;
    end

== matlab function Model_turn/LIMB 1: Back LEFT/Limb 1/MATLAB Function2 ==
  data: R input; roll_deg output; pitch_deg output; yaw_deg output
function [roll_deg, pitch_deg, yaw_deg] = orientation_to_plane_angles(R)
    roll = atan2(R(3,2), R(3,3));
    pitch = asin(-R(3,1));
    yaw = atan2(R(2,1), R(1,1));
    % Convert angles from radians to degrees
    roll_deg = rad2deg(roll);
    pitch_deg = rad2deg(pitch);
    yaw_deg = rad2deg(yaw);

end

== matlab function Model_turn/LIMB 1: Center LEFT/Limb 1/SMA2 F(V)/F(T) ==
  data: T input; F output; Fmax_SMA input
function F = fcn(T, Fmax_SMA)

% INPUT: Temperature (C), max SMA force
% OUTPUT: Force [N]

% Based around T_transition = 90C

% THOS WHOLE RELATIONSHIP NEEDS IMPROVEMENT, LOOSELY BASED ON fig 6b from:
% https://link.springer.com/article/10.1007/s11340-024-01059-9 and 
% https://www.dynalloy.com/pdfs/TCF1140_2.pdf
if T>110
    F = Fmax_SMA;
elseif T>95
    F = Fmax_SMA - 0.2*Fmax_SMA * ((110-T)/15);
elseif T>85
    F = 0.8*Fmax_SMA - 0.55*Fmax_SMA * ((95-T)/10);
else
    F = 0.25*Fmax_SMA - 0.25*Fmax_SMA * ((85-T)/50);
end

== matlab function Model_turn/LIMB 1: Back LEFT/Limb 1/SMA1 F(V)/F(T) ==
  data: T input; F output; Fmax_SMA input
function F = fcn(T, Fmax_SMA)

% INPUT: Temperature (C), max SMA force
% OUTPUT: Force [N]

% Based around T_transition = 90C

% THOS WHOLE RELATIONSHIP NEEDS IMPROVEMENT, LOOSELY BASED ON fig 6b from:
% https://link.springer.com/article/10.1007/s11340-024-01059-9 and 
% https://www.dynalloy.com/pdfs/TCF1140_2.pdf
if T>110
    F = Fmax_SMA;
elseif T>95
    F = Fmax_SMA - 0.2*Fmax_SMA * ((110-T)/15);
elseif T>85
    F = 0.8*Fmax_SMA - 0.55*Fmax_SMA * ((95-T)/10);
else
    F = 0.25*Fmax_SMA - 0.25*Fmax_SMA * ((85-T)/50);
end

== matlab function Model_turn/LIMB 1: Back LEFT/Limb 1/SMA2 F(V)/F(T) ==
  data: T input; F output; Fmax_SMA input
function F = fcn(T, Fmax_SMA)

% INPUT: Temperature (C), max SMA force
% OUTPUT: Force [N]

% Based around T_transition = 90C

% THOS WHOLE RELATIONSHIP NEEDS IMPROVEMENT, LOOSELY BASED ON fig 6b from:
% https://link.springer.com/article/10.1007/s11340-024-01059-9 and 
% https://www.dynalloy.com/pdfs/TCF1140_2.pdf
if T>110
    F = Fmax_SMA;
elseif T>95
    F = Fmax_SMA - 0.2*Fmax_SMA * ((110-T)/15);
elseif T>85
    F = 0.8*Fmax_SMA - 0.55*Fmax_SMA * ((95-T)/10);
else
    F = 0.25*Fmax_SMA - 0.25*Fmax_SMA * ((85-T)/50);
end

== matlab function Model_turn/LIMB 1: Back LEFT/Limb 1/SMA3 F(V)/F(T) ==
  data: T input; F output; Fmax_SMA input
function F = fcn(T, Fmax_SMA)

% INPUT: Temperature (C), max SMA force
% OUTPUT: Force [N]

% Based around T_transition = 90C

% THOS WHOLE RELATIONSHIP NEEDS IMPROVEMENT, LOOSELY BASED ON fig 6b from:
% https://link.springer.com/article/10.1007/s11340-024-01059-9 and 
% https://www.dynalloy.com/pdfs/TCF1140_2.pdf
if T>110
    F = Fmax_SMA;
elseif T>95
    F = Fmax_SMA - 0.2*Fmax_SMA * ((110-T)/15);
elseif T>85
    F = 0.8*Fmax_SMA - 0.55*Fmax_SMA * ((95-T)/10);
else
    F = 0.25*Fmax_SMA - 0.25*Fmax_SMA * ((85-T)/50);
end

== matlab function Model_turn/LIMB 1: Back LEFT/Limb 1/SMA4 F(V)/F(T) ==
  data: T input; F output; Fmax_SMA input
function F = fcn(T, Fmax_SMA)

% INPUT: Temperature (C), max SMA force
% OUTPUT: Force [N]

% Based around T_transition = 90C

% THOS WHOLE RELATIONSHIP NEEDS IMPROVEMENT, LOOSELY BASED ON fig 6b from:
% https://link.springer.com/article/10.1007/s11340-024-01059-9 and 
% https://www.dynalloy.com/pdfs/TCF1140_2.pdf
if T>110
    F = Fmax_SMA;
elseif T>95
    F = Fmax_SMA - 0.2*Fmax_SMA * ((110-T)/15);
elseif T>85
    F = 0.8*Fmax_SMA - 0.55*Fmax_SMA * ((95-T)/10);
else
    F = 0.25*Fmax_SMA - 0.25*Fmax_SMA * ((85-T)/50);
end

== matlab function Model_turn/LIMB 1: Back LEFT/PID CONTROLLER ==
  data: eX input; deX input; seX input; D1 output; eY input; D2 output; D3 output; D4 output; deY input; seY input; PWM_max input
function [D1, D2, D3, D4] = fcn(eX, deX, seX, eY, deY, seY, PWM_max)

    % INPUT: errors and derivatives about -x and -y axes, max PWM
    % OUTPUT: Duty Cycles:

    kp = 0.5;
    kd = 0;
    ki = 0.05;

    D1 = 0; D2 = 0; D3 = 0; D4 = 0;

    if eX > 0.5
        D1 = min((kp*eX + kd*deX + ki*seX), PWM_max);
    elseif eX < -0.5
        D2 = min((kp*-eX + kd*-deX + ki*-seX), PWM_max);
    end

    if eY > 0.5
        D3 = min((kp*eY + kd*deY + ki*seY), PWM_max);
    elseif eY < -0.5
        D4 = min((kp*-eY + kd*-deY + ki*-seY), PWM_max);
    end

== matlab function Model_turn/LIMB 1: Center RIGHT/BANG-BANG CONTROLLER ==
  data: theta_X input; D1 output; theta_Y input; D2 output; D3 output; D4 output; Target_X input; Target_Y input; PWM_max input
function [D1, D2, D3, D4] = fcn(theta_X, theta_Y, Target_X, Target_Y, PWM_max)

    % INPUT: Rotations about -X and -Y axes, Target angles, max PWM
    % OUTPUT: Duty Cycles:
    %   D1: +X rotation
    %   D2: -X rotation
    %   D3: +Y rotation
    %   D4: -Y rotation

    X_err = Target_X - theta_X;
    Y_err = Target_Y - theta_Y;

    D1 = 0; D2 = 0; D3 = 0; D4 = 0;

    if X_err > 5
        D1 = PWM_max;
    elseif X_err > 1
        D1 = PWM_max / 1.5;
    elseif X_err < -5
        D2 = PWM_max;
    elseif X_err < -1
        D2 = PWM_max / 1.5;
    end

    if Y_err > 5
        D3 = PWM_max;
    elseif Y_err > 1
        D3 = PWM_max / 1.5;
    elseif Y_err < -5
        D4 = PWM_max;
    elseif Y_err < -1
        D4 = PWM_max / 1.5;
    end

== matlab function Model_turn/LIMB 1: Center RIGHT/Limb 1/MATLAB Function2 ==
  data: R input; roll_deg output; pitch_deg output; yaw_deg output
function [roll_deg, pitch_deg, yaw_deg] = orientation_to_plane_angles(R)
    roll = atan2(R(3,2), R(3,3));
    pitch = asin(-R(3,1));
    yaw = atan2(R(2,1), R(1,1));
    % Convert angles from radians to degrees
    roll_deg = rad2deg(roll);
    pitch_deg = rad2deg(pitch);
    yaw_deg = rad2deg(yaw);

end

== matlab function Model_turn/LIMB 1: Center RIGHT/Limb 1/SMA1 F(V)/F(T) ==
  data: T input; F output; Fmax_SMA input
function F = fcn(T, Fmax_SMA)

% INPUT: Temperature (C), max SMA force
% OUTPUT: Force [N]

% Based around T_transition = 90C

% THOS WHOLE RELATIONSHIP NEEDS IMPROVEMENT, LOOSELY BASED ON fig 6b from:
% https://link.springer.com/article/10.1007/s11340-024-01059-9 and 
% https://www.dynalloy.com/pdfs/TCF1140_2.pdf
if T>110
    F = Fmax_SMA;
elseif T>95
    F = Fmax_SMA - 0.2*Fmax_SMA * ((110-T)/15);
elseif T>85
    F = 0.8*Fmax_SMA - 0.55*Fmax_SMA * ((95-T)/10);
else
    F = 0.25*Fmax_SMA - 0.25*Fmax_SMA * ((85-T)/50);
end

== matlab function Model_turn/LIMB 1: Center LEFT/Limb 1/SMA1 F(V)/F(T) ==
  data: T input; F output; Fmax_SMA input
function F = fcn(T, Fmax_SMA)

% INPUT: Temperature (C), max SMA force
% OUTPUT: Force [N]

% Based around T_transition = 90C

% THOS WHOLE RELATIONSHIP NEEDS IMPROVEMENT, LOOSELY BASED ON fig 6b from:
% https://link.springer.com/article/10.1007/s11340-024-01059-9 and 
% https://www.dynalloy.com/pdfs/TCF1140_2.pdf
if T>110
    F = Fmax_SMA;
elseif T>95
    F = Fmax_SMA - 0.2*Fmax_SMA * ((110-T)/15);
elseif T>85
    F = 0.8*Fmax_SMA - 0.55*Fmax_SMA * ((95-T)/10);
else
    F = 0.25*Fmax_SMA - 0.25*Fmax_SMA * ((85-T)/50);
end

== matlab function Model_turn/LIMB 1: Center RIGHT/Limb 1/SMA2 F(V)/F(T) ==
  data: T input; F output; Fmax_SMA input
function F = fcn(T, Fmax_SMA)

% INPUT: Temperature (C), max SMA force
% OUTPUT: Force [N]

% Based around T_transition = 90C

% THOS WHOLE RELATIONSHIP NEEDS IMPROVEMENT, LOOSELY BASED ON fig 6b from:
% https://link.springer.com/article/10.1007/s11340-024-01059-9 and 
% https://www.dynalloy.com/pdfs/TCF1140_2.pdf
if T>110
    F = Fmax_SMA;
elseif T>95
    F = Fmax_SMA - 0.2*Fmax_SMA * ((110-T)/15);
elseif T>85
    F = 0.8*Fmax_SMA - 0.55*Fmax_SMA * ((95-T)/10);
else
    F = 0.25*Fmax_SMA - 0.25*Fmax_SMA * ((85-T)/50);
end

== matlab function Model_turn/LIMB 1: Center RIGHT/Limb 1/SMA3 F(V)/F(T) ==
  data: T input; F output; Fmax_SMA input
function F = fcn(T, Fmax_SMA)

% INPUT: Temperature (C), max SMA force
% OUTPUT: Force [N]

% Based around T_transition = 90C

% THOS WHOLE RELATIONSHIP NEEDS IMPROVEMENT, LOOSELY BASED ON fig 6b from:
% https://link.springer.com/article/10.1007/s11340-024-01059-9 and 
% https://www.dynalloy.com/pdfs/TCF1140_2.pdf
if T>110
    F = Fmax_SMA;
elseif T>95
    F = Fmax_SMA - 0.2*Fmax_SMA * ((110-T)/15);
elseif T>85
    F = 0.8*Fmax_SMA - 0.55*Fmax_SMA * ((95-T)/10);
else
    F = 0.25*Fmax_SMA - 0.25*Fmax_SMA * ((85-T)/50);
end

== matlab function Model_turn/LIMB 1: Center RIGHT/Limb 1/SMA4 F(V)/F(T) ==
  data: T input; F output; Fmax_SMA input
function F = fcn(T, Fmax_SMA)

% INPUT: Temperature (C), max SMA force
% OUTPUT: Force [N]

% Based around T_transition = 90C

% THOS WHOLE RELATIONSHIP NEEDS IMPROVEMENT, LOOSELY BASED ON fig 6b from:
% https://link.springer.com/article/10.1007/s11340-024-01059-9 and 
% https://www.dynalloy.com/pdfs/TCF1140_2.pdf
if T>110
    F = Fmax_SMA;
elseif T>95
    F = Fmax_SMA - 0.2*Fmax_SMA * ((110-T)/15);
elseif T>85
    F = 0.8*Fmax_SMA - 0.55*Fmax_SMA * ((95-T)/10);
else
    F = 0.25*Fmax_SMA - 0.25*Fmax_SMA * ((85-T)/50);
end

== matlab function Model_turn/LIMB 1: Center RIGHT/PID CONTROLLER ==
  data: eX input; deX input; seX input; D1 output; eY input; D2 output; D3 output; D4 output; deY input; seY input; PWM_max input
function [D1, D2, D3, D4] = fcn(eX, deX, seX, eY, deY, seY, PWM_max)

    % INPUT: errors and derivatives about -x and -y axes, max PWM
    % OUTPUT: Duty Cycles:

    kp = 0.5;
    kd = 0;
    ki = 0.05;

    D1 = 0; D2 = 0; D3 = 0; D4 = 0;

    if eX > 0.5
        D1 = min((kp*eX + kd*deX + ki*seX), PWM_max);
    elseif eX < -0.5
        D2 = min((kp*-eX + kd*-deX + ki*-seX), PWM_max);
    end

    if eY > 0.5
        D3 = min((kp*eY + kd*deY + ki*seY), PWM_max);
    elseif eY < -0.5
        D4 = min((kp*-eY + kd*-deY + ki*-seY), PWM_max);
    end

== matlab function Model_turn/LIMB 1: Front RIGHT/BANG-BANG CONTROLLER ==
  data: theta_X input; D1 output; theta_Y input; D2 output; D3 output; D4 output; Target_X input; Target_Y input; PWM_max input
function [D1, D2, D3, D4] = fcn(theta_X, theta_Y, Target_X, Target_Y, PWM_max)

    % INPUT: Rotations about -X and -Y axes, Target angles, max PWM
    % OUTPUT: Duty Cycles:
    %   D1: +X rotation
    %   D2: -X rotation
    %   D3: +Y rotation
    %   D4: -Y rotation

    X_err = Target_X - theta_X;
    Y_err = Target_Y - theta_Y;

    D1 = 0; D2 = 0; D3 = 0; D4 = 0;

    if X_err > 5
        D1 = PWM_max;
    elseif X_err > 1
        D1 = PWM_max / 1.5;
    elseif X_err < -5
        D2 = PWM_max;
    elseif X_err < -1
        D2 = PWM_max / 1.5;
    end

    if Y_err > 5
        D3 = PWM_max;
    elseif Y_err > 1
        D3 = PWM_max / 1.5;
    elseif Y_err < -5
        D4 = PWM_max;
    elseif Y_err < -1
        D4 = PWM_max / 1.5;
    end

== matlab function Model_turn/LIMB 1: Front RIGHT/Limb 1/MATLAB Function2 ==
  data: R input; roll_deg output; pitch_deg output; yaw_deg output
function [roll_deg, pitch_deg, yaw_deg] = orientation_to_plane_angles(R)
    roll = atan2(R(3,2), R(3,3));
    pitch = asin(-R(3,1));
    yaw = atan2(R(2,1), R(1,1));
    % Convert angles from radians to degrees
    roll_deg = rad2deg(roll);
    pitch_deg = rad2deg(pitch);
    yaw_deg = rad2deg(yaw);

end

== matlab function Model_turn/LIMB 1: Front RIGHT/Limb 1/SMA1 F(V)/F(T) ==
  data: T input; F output; Fmax_SMA input
function F = fcn(T, Fmax_SMA)

% INPUT: Temperature (C), max SMA force
% OUTPUT: Force [N]

% Based around T_transition = 90C

% THOS WHOLE RELATIONSHIP NEEDS IMPROVEMENT, LOOSELY BASED ON fig 6b from:
% https://link.springer.com/article/10.1007/s11340-024-01059-9 and 
% https://www.dynalloy.com/pdfs/TCF1140_2.pdf
if T>110
    F = Fmax_SMA;
elseif T>95
    F = Fmax_SMA - 0.2*Fmax_SMA * ((110-T)/15);
elseif T>85
    F = 0.8*Fmax_SMA - 0.55*Fmax_SMA * ((95-T)/10);
else
    F = 0.25*Fmax_SMA - 0.25*Fmax_SMA * ((85-T)/50);
end

== matlab function Model_turn/LIMB 1: Front RIGHT/Limb 1/SMA2 F(V)/F(T) ==
  data: T input; F output; Fmax_SMA input
function F = fcn(T, Fmax_SMA)

% INPUT: Temperature (C), max SMA force
% OUTPUT: Force [N]

% Based around T_transition = 90C

% THOS WHOLE RELATIONSHIP NEEDS IMPROVEMENT, LOOSELY BASED ON fig 6b from:
% https://link.springer.com/article/10.1007/s11340-024-01059-9 and 
% https://www.dynalloy.com/pdfs/TCF1140_2.pdf
if T>110
    F = Fmax_SMA;
elseif T>95
    F = Fmax_SMA - 0.2*Fmax_SMA * ((110-T)/15);
elseif T>85
    F = 0.8*Fmax_SMA - 0.55*Fmax_SMA * ((95-T)/10);
else
    F = 0.25*Fmax_SMA - 0.25*Fmax_SMA * ((85-T)/50);
end

== matlab function Model_turn/LIMB 1: Center LEFT/Limb 1/SMA3 F(V)/F(T) ==
  data: T input; F output; Fmax_SMA input
function F = fcn(T, Fmax_SMA)

% INPUT: Temperature (C), max SMA force
% OUTPUT: Force [N]

% Based around T_transition = 90C

% THOS WHOLE RELATIONSHIP NEEDS IMPROVEMENT, LOOSELY BASED ON fig 6b from:
% https://link.springer.com/article/10.1007/s11340-024-01059-9 and 
% https://www.dynalloy.com/pdfs/TCF1140_2.pdf
if T>110
    F = Fmax_SMA;
elseif T>95
    F = Fmax_SMA - 0.2*Fmax_SMA * ((110-T)/15);
elseif T>85
    F = 0.8*Fmax_SMA - 0.55*Fmax_SMA * ((95-T)/10);
else
    F = 0.25*Fmax_SMA - 0.25*Fmax_SMA * ((85-T)/50);
end

== matlab function Model_turn/LIMB 1: Front RIGHT/Limb 1/SMA3 F(V)/F(T) ==
  data: T input; F output; Fmax_SMA input
function F = fcn(T, Fmax_SMA)

% INPUT: Temperature (C), max SMA force
% OUTPUT: Force [N]

% Based around T_transition = 90C

% THOS WHOLE RELATIONSHIP NEEDS IMPROVEMENT, LOOSELY BASED ON fig 6b from:
% https://link.springer.com/article/10.1007/s11340-024-01059-9 and 
% https://www.dynalloy.com/pdfs/TCF1140_2.pdf
if T>110
    F = Fmax_SMA;
elseif T>95
    F = Fmax_SMA - 0.2*Fmax_SMA * ((110-T)/15);
elseif T>85
    F = 0.8*Fmax_SMA - 0.55*Fmax_SMA * ((95-T)/10);
else
    F = 0.25*Fmax_SMA - 0.25*Fmax_SMA * ((85-T)/50);
end

== matlab function Model_turn/LIMB 1: Front RIGHT/Limb 1/SMA4 F(V)/F(T) ==
  data: T input; F output; Fmax_SMA input
function F = fcn(T, Fmax_SMA)

% INPUT: Temperature (C), max SMA force
% OUTPUT: Force [N]

% Based around T_transition = 90C

% THOS WHOLE RELATIONSHIP NEEDS IMPROVEMENT, LOOSELY BASED ON fig 6b from:
% https://link.springer.com/article/10.1007/s11340-024-01059-9 and 
% https://www.dynalloy.com/pdfs/TCF1140_2.pdf
if T>110
    F = Fmax_SMA;
elseif T>95
    F = Fmax_SMA - 0.2*Fmax_SMA * ((110-T)/15);
elseif T>85
    F = 0.8*Fmax_SMA - 0.55*Fmax_SMA * ((95-T)/10);
else
    F = 0.25*Fmax_SMA - 0.25*Fmax_SMA * ((85-T)/50);
end

== matlab function Model_turn/LIMB 1: Front RIGHT/PID CONTROLLER ==
  data: eX input; deX input; seX input; D1 output; eY input; D2 output; D3 output; D4 output; deY input; seY input; PWM_max input
function [D1, D2, D3, D4] = fcn(eX, deX, seX, eY, deY, seY, PWM_max)

    % INPUT: errors and derivatives about -x and -y axes, max PWM
    % OUTPUT: Duty Cycles:

    kp = 0.5;
    kd = 0;
    ki = 0.05;

    D1 = 0; D2 = 0; D3 = 0; D4 = 0;

    if eX > 0.5
        D1 = min((kp*eX + kd*deX + ki*seX), PWM_max);
    elseif eX < -0.5
        D2 = min((kp*-eX + kd*-deX + ki*-seX), PWM_max);
    end

    if eY > 0.5
        D3 = min((kp*eY + kd*deY + ki*seY), PWM_max);
    elseif eY < -0.5
        D4 = min((kp*-eY + kd*-deY + ki*-seY), PWM_max);
    end

== matlab function Model_turn/MATLAB Function ==
  data: p0 input; xfl output; yfl output; xcl output; ycl output; xbl output; ybl output; xfr output; yfr output; xcr output; ycr output; xbr output; ybr output; p1 input; p2 input; p3 input; p4 input; p5 input; p6 input; p7 input; swing_angle input
function [xfl, yfl, xcl, ycl, xbl, ybl, xfr, yfr, xcr, ycr, xbr, ybr]= turn(p0, p1, p2, p3, p4, p5, p6, p7, swing_angle)


in = 20;
out = 30;
forward = swing_angle;
backward = -swing_angle;

if (p0 == 1) % start
    xfl = 0;
    xbl = 0;
    xcr = 0;
    xcl = 0;
    xfr = 0;
    xbr = 0;
    yfl = 0;
    ybl = 0;
    ycr = 0;
    ycl = 0;
    yfr = 0;
    ybr = 0;

elseif (p1 == 1) % legs out
    xfl = 0;
    xbl = 0;
    xcr = 0;
    xcl = 0;
    xfr = 0;
    xbr = 0;
    yfl = -in;
    ybl = -in;
    ycr = in;
    ycl = out;
    yfr = -out;
    ybr = -out;


elseif (p2 == 1) % legs out and forward/back
    xfl = backward;
    xbl = backward;
    xcr = forward;
    xcl = forward;
    xfr = backward;
    xbr = backward;
    yfl = -in;
    ybl = -in;
    ycr = in;
    ycl = out;
    yfr = -out;
    ybr = -out;

elseif (p3 == 1) % stand again
    xfl = backward;
    xbl = backward;
    xcr = forward;
    xcl = forward;
    xfr = backward;
    xbr = backward;
    yfl = -in;
    ybl = -in;
    ycr = in;
    ycl = -in;
    yfr = in;
    ybr = in;

elseif (p4 == 1) % lift other legs
    xfl = backward;
    xbl = backward;
    xcr = forward;
    xcl = forward;
    xfr = backward;
    xbr = backward;
    yfl = out;
    ybl = out;
    ycr = -out;
    ycl = -in;
    yfr = in;
    ybr = in;

elseif (p5 == 1) % move forward
    xfl = forward;
    xbl = forward;
    xcr = backward;
    xcl = backward;
    xfr = forward;
    xbr = forward;
    yfl = out;
    ybl = out;
    ycr = -out;
    ycl = -in;
    yfr = in;
    ybr = in;

elseif (p6 == 1) % stand again
    xfl = forward;
    xbl = forward;
    xcr = backward;
    xcl = backward;
    xfr = forward;
    xbr = forward;
    yfl = -in;
    ybl = -in;
    ycr = in;
    ycl = -in;
    yfr = in;
    ybr = in;   

elseif(p7 ==1) % replaces p1 in loop
    xfl = forward;
    xbl = forward;
    xcr = backward;
    xcl = backward;
    xfr = forward;
    xbr = forward;
    yfl = -in;
    ybl = -in;
    ycr = in;
    ycl = out;
    yfr = -out;
    ybr = -out;
else
    xfl = 0;
    xbl = 0;
    xcr = 0;
    xcl = 0;
    xfr = 0;
    xbr = 0;
    yfl = 0;
    ybl = 0;
    ycr = 0;
    ycl = 0;
    yfr = 0;
    ybr = 0;
end



% xfl = 0;
% xbl = 0;
% xcr = 0;
% xcl = 0;
% xfr = 0;
% xbr = 0;
% yfl = -10;
% ybl = -10;
% ycr = 0;
% ycl = 30;
% yfr = -30;
% ybr = -30;
